simulink subsystem "test_received_frames"  (R2024b)
settings: Solver=VariableStepAuto  StartTime=0.0  StopTime=10.0  RelTol=1e-3
undefined symbols (not defined in the file): Param
libraries: commsink2 x1
settings Model: Creator=SERGIO  LastModifiedBy=rober

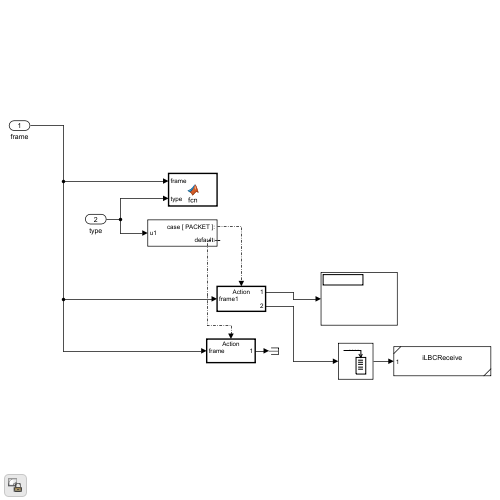
[thumbnail: Simulink's stored preview of the top-level diagram]
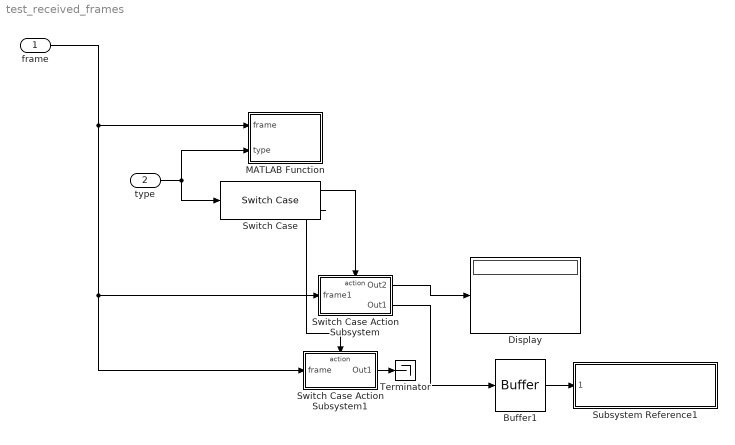
== system test_received_frames ==
  frame : Inport
  type : Inport  Port=2
  Buffer1 : Buffer  N=400  OutputFrames=off
  Display : Display
  MATLAB Function : MATLAB Function  TreatAsAtomicUnit=on
  Subsystem Reference1 : Subsystem  ReferencedSubsystem=iLBCReceive
  Switch Case : SwitchCase  CaseConditions={frameType.PACKET}
  Switch Case Action Subsystem : Subsystem  TreatAsAtomicUnit=on
  Switch Case Action Subsystem1 : Subsystem  TreatAsAtomicUnit=on
  Terminator : Terminator
  wires:
  frame/1 -> Switch Case Action Subsystem1/1(frame), Switch Case Action Subsystem/1(frame1), MATLAB Function/1(frame)
  type/1 -> Switch Case/1, MATLAB Function/2(type)
  Switch Case/1 -> Switch Case Action Subsystem/Action
  Switch Case Action Subsystem/1(Out2) -> Display/1
  Switch Case/2 -> Switch Case Action Subsystem1/Action
  Buffer1/1 -> Subsystem Reference1/1
  Switch Case Action Subsystem/2(Out1) -> Buffer1/1
  Switch Case Action Subsystem1/1(Out1) -> Terminator/1

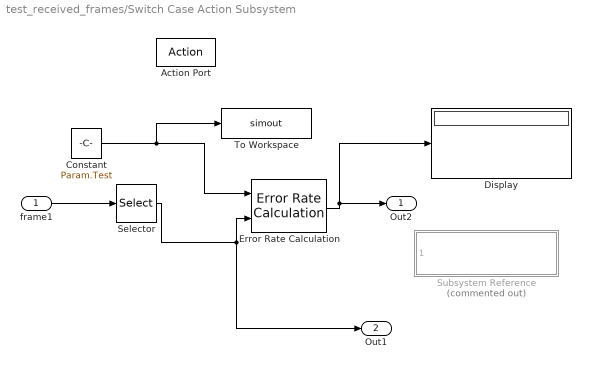
== system test_received_frames/Switch Case Action Subsystem ==
  frame1 : Inport
  Action Port : ActionPort
  Constant : Constant  Value=Param.Test  VectorParams1D=off
  Display : Display
  Error Rate Calculation : commsink2/Error Rate Calculation  N=0  st_delay=0  cp_mode=Entire frame  subframe=[]  PMode=Port  WsName=ErrorVec  RsMode2=off  stop=off  numErr=100  maxBits=1e6
  Selector : Selector  IndexOptions=Index vector (dialog)  Indices=[1:200]  OutputSizes=1
  Subsystem Reference : Subsystem  Commented=on  ReferencedSubsystem=AudioRecive
  To Workspace : ToWorkspace  VariableName=simout  SampleTime=-1
      settings: Save2DSignal=2-D array (concatenate along first dimension)
  Out2 : Outport
  Out1 : Outport  Port=2
  wires:
  Error Rate Calculation/1 -> Out2/1, Display/1
  frame1/1 -> Selector/1
  Constant/1 -> To Workspace/1, Error Rate Calculation/1
  Selector/1 -> Error Rate Calculation/2, Out1/1

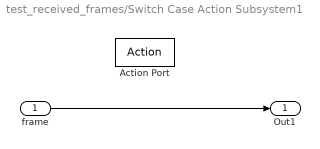
== system test_received_frames/Switch Case Action Subsystem1 ==
  frame : Inport
  Action Port : ActionPort
  Out1 : Outport
  wires:
  frame/1 -> Out1/1

== matlab function test_received_frames/MATLAB Function ==
  data: frame input; type input
function fcn(frame, type)

if type == frameType.LSF
    fprintf("%s","Received LSF correctly")
elseif type == frameType.PACKET
    fprintf("%s","Received Packet correctly")
elseif type == frameType.INVALID
    fprintf("%s", "Nothing")
end
